simulink model "sf_stickslip"  (Simulink 6.0)
settings: Solver=ode15s  SolverMode=SingleTasking  StartTime=0.0  StopTime=20  RelTol=1e-3  AbsTol=1e-6
PreLoadFcn:
  | load('sf_stickslipdat')
values from neighbouring files (symbols this model uses):
  Fsliding = 1    [sf_electrohydraulic.mat]    (also in sf_stickslipdat.mat)
  Fstatic = 1    [sf_electrohydraulic.mat]    (also in sf_stickslipdat.mat)
  K = 1    [sf_stickslipdat.mat]
  M = 0.001    [sf_stickslipdat.mat]
libraries: simulink x1
settings Model: CovMetricSettings=dcmtr  Creator=The MathWorks Inc.  LastModifiedBy=batserve  ExtModeTrigMode=oneshot  ExtModeArmWhenConnect=off  ExtModeAutoUpdateStatusClock=off
settings DataIOCC: LimitDataPoints=off  SaveState=on
settings OptimizationCC: BooleanDataType=off
settings DebuggingCC: CheckExecutionContextPreStartOutputMsg=on  CheckExecutionContextRuntimeOutputMsg=on  SolverPrmCheckMsg=none  IntegerOverflowMsg=none
settings HardwareCC: TargetUnknown=on

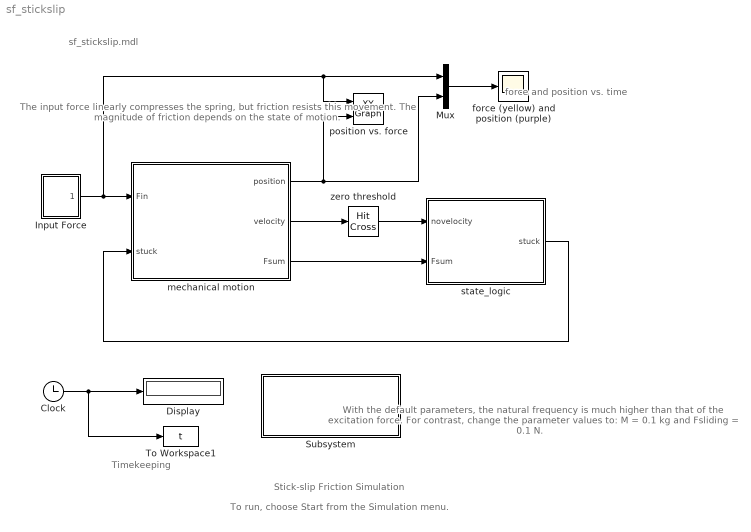
== system sf_stickslip ==
  note: The input force linearly compresses
      | the spring, but friction resists this
      | movement.  The magnitude of
      | friction depends on the state of motion.
  note: force and
      | position
      | vs. time
  note: With the default parameters, the natural
      | frequency is much higher than that of the
      | excitation force.  For contrast, change
      | the parameter values to:
      | M = 0.1 kg and Fsliding = 0.1 N.
  note: Stick-slip Friction Simulation
  note: sf_stickslip.mdl
  note: Timekeeping
  note: To run, choose Start from the Simulation menu.
  Clock : Clock
      settings: Decimation=10
  Display : Display
  Input Force : Subsystem  PropExecContextAcrossSSBoundary=on  mask(Repeating table){rep_seq_t=[0 5 10], rep_seq_y=[0 5 0]}
      mask prompts: rep_seq_t "Time values:"; rep_seq_y "Output values:"
      mask help: Repeating table.
      mask init:
      | period = max(rep_seq_t);
      mask Help: Repeats cycle given in table. Time values should be monotonically increasing.
      mask Display: plot([rep_seq_t,rep_seq_t+period,rep_seq_t+2*period,rep_seq_t(1)+3*period],[rep_seq_y,rep_seq_y,rep_seq_y,rep_seq_y(1)])
  Mux : Mux  Inputs=2
  Subsystem : Subsystem  PropExecContextAcrossSSBoundary=on
      settings: OpenFcn=sf_stickslipedit
      mask Display: disp('edit\nparameters')
  To Workspace1 : ToWorkspace  VariableName=t  SampleTime=-1  SaveFormat=Array
  force (yellow) and position (purple) : Scope
      settings: TickLabels=on  YMax=10  DataFormat=Array
  mechanical motion : Subsystem  PropExecContextAcrossSSBoundary=on
      mask Display:
      | plot(-2,-1,7,3,[0 5],[0 0],[1 1 3 3],[0 2 2 0],[4.5 4.5],[0 3.5],[3 3.25 3.5 3.75 4 4.25 4.5], [1 1 .5  1.5  .5 1 1],[0 1],[1 1],[.5 1 .5],[.5 1 1.5],
      | [0 .5],[-.5 0],[1 1.5],[-.5 0],[2 2.5],[-.5 0],[3 3.5],[-.5 0],[4 5],[-.5 .5],
      | [4.5 5],[1 1.5],[4.5 5],[2 2.5],[4.5 5],[3 3.5],[max(-0.5:0.5:2.5, 1);min(1.5:0.5:4.5,3)],[min(0.5:0.5:3.5, 2); max(-1.5:0.5:1.5, 0)])
  position vs. force : simulink/Sinks/XY Graph  xmin=-1  xmax=6  ymin=-1  ymax=6  st=-1
  state_logic : Stateflow chart  PropExecContextAcrossSSBoundary=on
  zero threshold : HitCross
  wires:
  Clock/1 -> Display/1, To Workspace1/1
  Mux/1 -> force (yellow) and position (purple)/1
  zero threshold/1 -> state_logic/1(novelocity)
  mechanical motion/3(Fsum) -> state_logic/2(Fsum)
  mechanical motion/2(velocity) -> zero threshold/1
  mechanical motion/1(position) -> Mux/2, position vs. force/2
  state_logic/1(stuck) -> mechanical motion/2(stuck)
  Input Force/1(out_1) -> mechanical motion/1(Fin), position vs. force/1, Mux/1

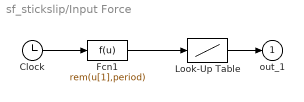
== system sf_stickslip/Input Force ==
  Clock : Clock
      settings: Decimation=10
  Fcn1 : Fcn  Expr=rem(u[1],period)
  Look-Up Table : Lookup  DialogController=Simulink.DDGSource  InputValues=rep_seq_t  OutputValues=rep_seq_y  SaturateOnIntegerOverflow=on
  out_1 : Outport  InitialOutput=0
  wires:
  Look-Up Table/1 -> out_1/1
  Clock/1 -> Fcn1/1
  Fcn1/1 -> Look-Up Table/1

== system sf_stickslip/Subsystem ==

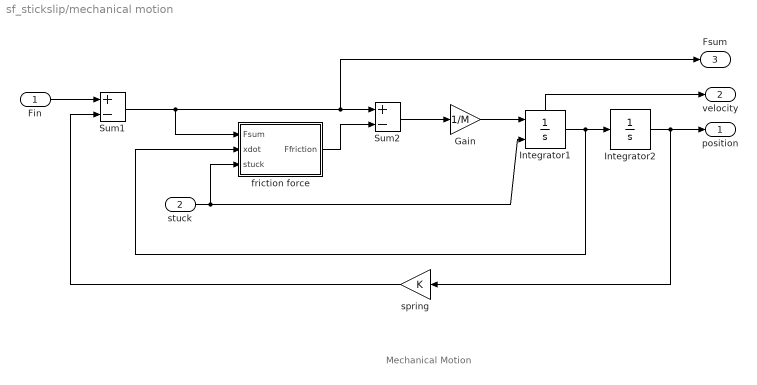
== system sf_stickslip/mechanical motion ==
  note: Mechanical Motion
  Fin : Inport  Port=1  LatchInput=off
  stuck : Inport  Port=2  LatchInput=off
  Gain : Gain  Gain=1/M  SaturateOnIntegerOverflow=on
  Integrator1 : Integrator  ExternalReset=rising  ShowStatePort=on
  Integrator2 : Integrator
  Sum1 : Sum  Inputs=+-  SaturateOnIntegerOverflow=on  InputSameDT=on
  Sum2 : Sum  Inputs=+-  SaturateOnIntegerOverflow=on  InputSameDT=on
  friction force : Subsystem  PropExecContextAcrossSSBoundary=on
  spring : Gain  Orientation=left  Gain=K  SaturateOnIntegerOverflow=on
  position : Outport  InitialOutput=0
  velocity : Outport  Port=2  InitialOutput=0
  Fsum : Outport  Port=3  InitialOutput=0
  wires:
  stuck/1 -> friction force/3(stuck), Integrator1/2
  Integrator1/1 -> friction force/2(xdot), Integrator2/1
  Gain/1 -> Integrator1/1
  spring/1 -> Sum1/2
  Sum1/1 -> friction force/1(Fsum), Sum2/1, Fsum/1
  Sum2/1 -> Gain/1
  friction force/1(Ffriction) -> Sum2/2
  Fin/1 -> Sum1/1
  Integrator1/State -> velocity/1
  Integrator2/1 -> spring/1, position/1

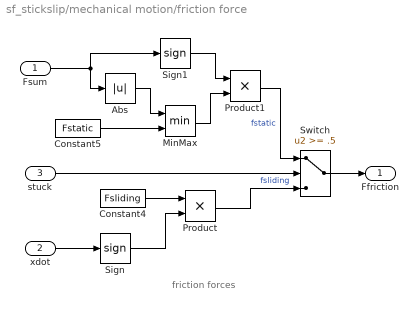
== system sf_stickslip/mechanical motion/friction force ==
  note: friction forces
  Fsum : Inport  Port=1  LatchInput=off
  xdot : Inport  Port=2  LatchInput=off
  stuck : Inport  Port=3  LatchInput=off
  Abs : Abs  SaturateOnIntegerOverflow=on
  Constant4 : Constant  Value=Fsliding
  Constant5 : Constant  Value=Fstatic
  MinMax : MinMax  Inputs=2  SaturateOnIntegerOverflow=on  InputSameDT=on
  Product : Product  SaturateOnIntegerOverflow=on  RndMeth=Zero  InputSameDT=on
  Product1 : Product  SaturateOnIntegerOverflow=on  RndMeth=Zero  InputSameDT=on
  Sign : Signum
  Sign1 : Signum
  Switch : Switch  Threshold=.5  SaturateOnIntegerOverflow=on  InputSameDT=on
  Ffriction : Outport  InitialOutput=0
  wires:
  Switch/1 -> Ffriction/1
  stuck/1 -> Switch/2
  xdot/1 -> Sign/1
  Sign/1 -> Product/2
  Product/1 -> Switch/3  "fsliding"
  Constant4/1 -> Product/1
  Sign1/1 -> Product1/1
  MinMax/1 -> Product1/2
  Constant5/1 -> MinMax/2
  Abs/1 -> MinMax/1
  Fsum/1 -> Sign1/1, Abs/1
  Product1/1 -> Switch/1  "fstatic"

== stateflow chart state_logic ==
  settings: updateMethod=CONTINUOUS
  state state_of_motion
    state stuck/
      entry: stuck = 1;
    state sliding/
      entry: stuck = 0;
    stuck -> sliding : [fabs(Fsum) > Fstatic]
    (default) -> stuck
    sliding -> stuck : [novelocity & (fabs(Fsum)<= Fstatic)]
  data: stuck output double [0..1]; novelocity input double; Fsum input double
  data stuck settings: units=int
